simulink model "servo_system_model"  (R2021a)
settings: Solver=FixedStepAuto  StartTime=0.0  StopTime=t_end  FixedStep=dt  RelTol=1e-3
values from neighbouring files (symbols this model uses):
  A = pi/16    (= 0.196349540849)    [control_design.m]
  b1 = 0.005    [simulation.m]
  b2 = 3.7e-6    (= 3.7e-06)    [simulation.m]
  dt = 1e-4    (= 0.0001)    [parameters.m]    (also in simulation.m)
  J1 = J_barra(1)/N1^2    [simulation.m]
  J2 = J_barra(2)/N2^2    [simulation.m]
  K_sensor = 12/(pi/4)    (= 15.2788745368)    [control_design.m]    (also in parameters.m; simulation.m)
  Kb1 = 0.018    [simulation.m]
  Kb2 = 0.0145    [simulation.m]
  Kd1 = 0    [simulation.m]
  Kd2 = 0    [simulation.m]
  Ki2 = 0    [simulation.m]
  Kp1 = 1, Ki1 = 0    [simulation.m]
  Kp2 = 1    [simulation.m]
  Kt1 = 0.018    [simulation.m]
  Kt2 = 0.0145    [simulation.m]
  La1 = 2.93e-3    (= 0.00293)    [simulation.m]
  La2 = 0.42e-3    (= 0.00042)    [simulation.m]
  m = p(1)    [control_design.m]
  mode = 1    [simulation.m]
  N = 5    [parameters.m]
  N1 = 5    [simulation.m]
  N2 = 15    [simulation.m]
  Ra1 = 0.89    [simulation.m]
  Ra2 = 0.7    [simulation.m]
  s = tf('s')    [control_design.m]
  sampling = 1    [simulation.m]
  theta1_ini = theta_m(1,1)    [parameters.m]    (also in simulation.m = -1.57079632679)
  theta2_ini = theta_m(2,1)    [parameters.m]    (also in simulation.m = 0)
undefined symbols (not defined in the file or in its folder): angle_ini, displacement, home, K, Ki1, L1, L2, m1, m2, phi, X, Y, Z
libraries: sm_lib x9, fl_lib x7, nesl_utility x7, ee_lib x5, pid_lib x3, simulink x1
settings Model: Creator=Juan_Cerquera  LastModifiedBy=Sebastian

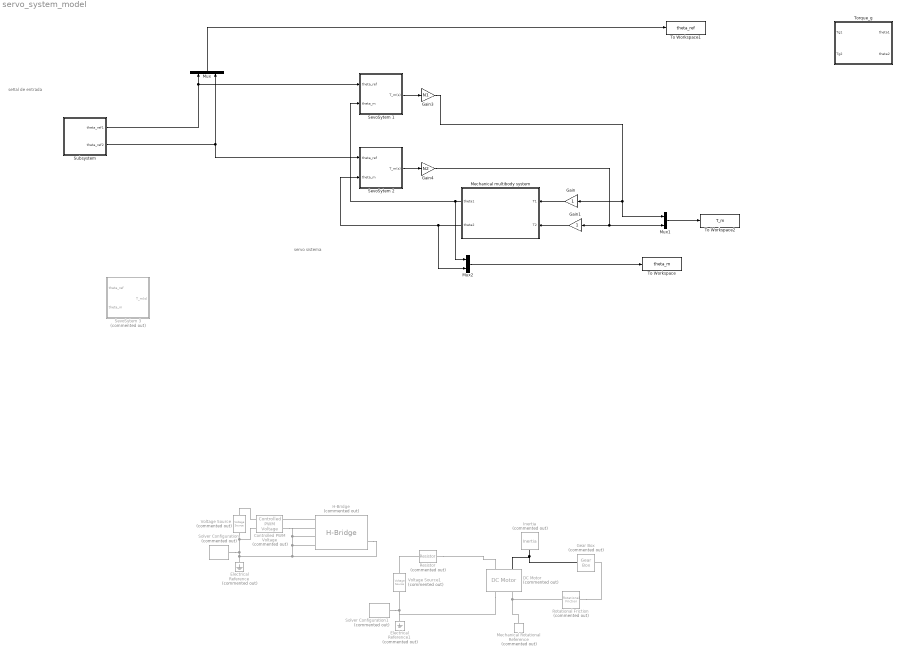
== system servo_system_model ==
  note: servo sistema
  note: señal de entrada
  Controlled PWM Voltage : ee_lib/Integrated Circuits/Controlled PWM Voltage  Commented=on  F=1000 Hz  TD=0 s  pulse_width_offset=0 s  pulse_min=0 s  Vmin=0 V  Vmax=5 V  Vm=5 V  pwm_or_av=2  event_type=1  sample_time=1e-6 s  u_min=0  u_max=1
  DC Motor : ee_lib/Electromechanical/Brushed Motors/DC Motor  Commented=on  field_option=ee.enum.field_option.pm  Rf=100 Ohm  Lf=1 H  Laf=0.15 H  If0=0 A  parameterization=ee.enum.dcparam_option.circuit_param  Ra=3.9 Ohm  La=12e-6 H  emf_or_torque=ee.enum.emf_or_torque.kv  Kv=0.072e-3 V/rpm  Ki=6.876e-4 N*m/A  T_stall=0.24e-3 N*m  w_max=19100 rpm  w_rated=15000 rpm  P_rated=0.08 W  V_rated=1.5 V  J=0.01 g*cm^2  lam_param=ee.enum.lam_param.damping  lam=0 N*m/(rad/s)  i_noload=0 A  V_i_noload=1.5 V  speed0=0 rpm  enable_fault_armature=ee.enum.faults.faultEnable.no  rev_faulted=1 / 3  G_faulted_armature=1e-5 S  fault_trigger_armature=ee.enum.faults.faultTrigger.temporal  t_fault_armature=1 s  max_permissible_current_armature=inf A  t_fail_on_current_armature=1 s  enable_fault_field=ee.enum.faults.faultEnable.no  G_faulted_field=1e-5 S  fault_trigger_field=ee.enum.faults.faultTrigger.temporal  t_fault_field=1 s  max_permissible_current_field=inf A  t_fail_on_current_field=1 s  fault_action=ee.enum.faults.faultAction.none  alpha=3.93e-3 1/K  Tmeas=25 degC  thermal_mass=100 J/K  initial_temperature=25 degC
  Electrical Reference : fl_lib/Electrical/Electrical Elements/Electrical Reference  Commented=on
  Electrical Reference1 : fl_lib/Electrical/Electrical Elements/Electrical Reference  Commented=on
  Gain : Gain
  Gain1 : Gain
  Gain3 : Gain  Gain=N1
  Gain4 : Gain  Gain=N2
  Gear Box : fl_lib/Mechanical/Mechanisms/Gear Box  Commented=on  ratio=5  t_in_specify=off  t_in_priority=None  t_in=0 N*m  t_in_nominal_specify=off  t_in_nominal_unit=N*m  t_in_nominal_value=1  t_out_specify=off  t_out_priority=None  t_out=0 N*m  t_out_nominal_specify=off  t_out_nominal_unit=N*m  t_out_nominal_value=1
  H-Bridge : ee_lib/Semiconductors & Converters/Converters/H-Bridge  Commented=on  supply_ports=ee.enum.supply_ports.hidesupply  Venable=2.5 V  Vmax=5.0 V  Vreverse=2.5 V  Vbrake=2.5 V  Vm=12 V  pwm_or_av=ee.enum.pwm_or_av.pwm  regenerative_braking_mode=ee.enum.converters.regenerative_braking_mode.depends_on_rev  discontinuous=ee.enum.current_profile.continuous  freewheeling_mode=ee.enum.converters.freewheeling_mode.one_switch_one_diode  Ron=0.1 Ohm  Don=0.05 Ohm  Goff=1e-6 S  Rload=10 Ohm  Lload=1e-5 H  F=10 kHz  thermal_mass=100 J/K  initial_temperature=298.15 K  Ron2=0.1 Ohm  Don2=0.05 Ohm  Tmeas=298.15 K  Tmeas2=398.15 K
  Inertia : fl_lib/Mechanical/Rotational Elements/Inertia  Commented=on  inertia=0.01 kg*m^2  num_ports=foundation.enum.numPorts2.one  w_specify=off  w_priority=High  w=0 rad/s  w_nominal_specify=off  w_nominal_unit=rad/s  w_nominal_value=1  t_specify=off  t_priority=None  t=0 N*m  t_nominal_specify=off  t_nominal_unit=N*m  t_nominal_value=1
  Mechanical Rotational Reference : fl_lib/Mechanical/Rotational Elements/Mechanical Rotational Reference  Commented=on
  "Mechanical multibody system " : Subsystem
  Mux : Mux  Inputs=2
  Mux1 : Mux  Inputs=2
  Mux2 : Mux  Inputs=2
  Resistor : fl_lib/Electrical/Electrical Elements/Resistor  Commented=on  R=1 Ohm  i_specify=off  i_priority=None  i=0 A  i_nominal_specify=off  i_nominal_unit=A  i_nominal_value=1  v_specify=off  v_priority=None  v=0 V  v_nominal_specify=off  v_nominal_unit=V  v_nominal_value=1
  Rotational Friction : fl_lib/Mechanical/Rotational Elements/Rotational Friction  Commented=on  brkwy_trq=25 N*m  brkwy_vel=0.1 rad/s  Col_trq=20 N*m  visc_coef=0.001 N*m/(rad/s)  w_specify=off  w_priority=None  w=0 rad/s  w_nominal_specify=off  w_nominal_unit=rad/s  w_nominal_value=1  t_specify=off  t_priority=None  t=0 N*m  t_nominal_specify=off  t_nominal_unit=N*m  t_nominal_value=1
  SevoSytem 1 : Subsystem  mask{P=Kp1, I=Ki1, D=Kd1, InitialCondition=theta1_ini, Electric=[La1 Ra1], Mechanic=[J1 b1], Kb=Kb1, Kt=Kt1, K_sensor=K_sensor}
      mask prompts: P "Simulink:masks:ProportionalP_MP"; I "Simulink:masks:IntegralI_MP"; D "Simulink:masks:DerivativeD_MP"; InitialCondition "Simulink:blkprm_prompts:AllBlksInitConds"; Electric "Electrical system Denominator"; Mechanic "Mechanical system Denominator"; Kb "Gain Kb:"; Kt "Gain Kt:"; K_sensor "Gain Sensor:"
      mask TypeOptions P: controlador/P
      mask TypeOptions I: controlador/I
      mask TypeOptions D: controlador/D
      mask TypeOptions InitialCondition: integrador/InitialCondition
      mask TypeOptions Electric: motor/Electric system/Denominator
      mask TypeOptions Mechanic: motor/Mechanic system/Denominator
      mask TypeOptions Kb: motor/kb/Gain
      mask TypeOptions Kt: motor/kt/Gain
      mask TypeOptions K_sensor: sensor/Gain
      mask DialogControl P Prompt: Proportional (P):
      mask DialogControl I Prompt: Integral (I):
      mask DialogControl D Prompt: Derivative (D):
      mask DialogControl InitialCondition Prompt: Initial conditions:
  SevoSytem 2 : Subsystem  mask{P=Kp2, I=Ki2, D=Kd2, InitialCondition=theta2_ini, Electric=[La2 Ra2], Mechanic=[J2 b2], Kb=Kb2, Kt=Kt2, K_sensor=K_sensor}
      mask prompts: P "Simulink:masks:ProportionalP_MP"; I "Simulink:masks:IntegralI_MP"; D "Simulink:masks:DerivativeD_MP"; InitialCondition "Simulink:blkprm_prompts:AllBlksInitConds"; Electric "Electrical system Denominator"; Mechanic "Mechanical system Denominator"; Kb "Gain Kb:"; Kt "Gain Kt:"; K_sensor "Gain Sensor:"
      mask TypeOptions P: controlador/P
      mask TypeOptions I: controlador/I
      mask TypeOptions D: controlador/D
      mask TypeOptions InitialCondition: integrador/InitialCondition
      mask TypeOptions Electric: motor/Electric system/Denominator
      mask TypeOptions Mechanic: motor/Mechanic system/Denominator
      mask TypeOptions Kb: motor/kb/Gain
      mask TypeOptions Kt: motor/kt/Gain
      mask TypeOptions K_sensor: sensor/Gain
      mask DialogControl P Prompt: Proportional (P):
      mask DialogControl I Prompt: Integral (I):
      mask DialogControl D Prompt: Derivative (D):
      mask DialogControl InitialCondition Prompt: Initial conditions:
  SevoSytem 3 : Subsystem  Commented=on  mask{P=Kp1, I=Ki1, D=Kd1, InitialCondition=theta1_ini, Electric=[La1 Ra1], Mechanic=[J1 b1], Kb=Kb1, Kt=Kt1, K_sensor=K_sensor}
      mask prompts: P "Simulink:masks:ProportionalP_MP"; I "Simulink:masks:IntegralI_MP"; D "Simulink:masks:DerivativeD_MP"; InitialCondition "Simulink:blkprm_prompts:AllBlksInitConds"; Electric "Electrical system Denominator"; Mechanic "Mechanical system Denominator"; Kb "Gain Kb:"; Kt "Gain Kt:"; K_sensor "Gain Sensor:"
      mask TypeOptions P: controlador/P
      mask TypeOptions I: controlador/I
      mask TypeOptions D: controlador/D
      mask TypeOptions InitialCondition: integrador/InitialCondition
      mask TypeOptions Electric: motor/Electric system/Denominator
      mask TypeOptions Mechanic: motor/Mechanic system/Denominator
      mask TypeOptions Kb: motor/kb/Gain
      mask TypeOptions Kt: motor/kt/Gain
      mask TypeOptions K_sensor: sensor/Gain
      mask DialogControl P Prompt: Proportional (P):
      mask DialogControl I Prompt: Integral (I):
      mask DialogControl D Prompt: Derivative (D):
      mask DialogControl InitialCondition Prompt: Initial conditions:
  Solver Configuration : nesl_utility/Solver Configuration  Commented=on  PhysicalDomain=network_engine_domain  SubClassName=solver  LeftPortType=input  RightPortType=generic  Tones=[]  Harmonics=[]  SimulateNoise=off  Profile=off  UseLocalSampling=off  EnableSwitchedLinearOptims=on  FrequencyDomain=off  UseCCode=off  RelTol=0.001  AbsTol=1e-06  MinStep=1e-09  ToWorkspace=off  RevertToSquareIcSolve=off  NumHomotopyIterations=100  PhasorMode=off  PhasorModeNumHarmonics=1  DoDC=off  ResidualTolerance=1e-09  UseLocalSolver=off  LocalSolverChoice=NE_BACKWARD_EULER_ADVANCER  LocalSolverSampleTime=0.001  DoFixedCost=off  MaxNonlinIter=3  MaxModeIter=2  ComputeImpulses=off  ImpulseIterations=2  LinearAlgebra=auto  EquationFormulation=NE_TIME_EF  DelaysMemoryBudget=1024  AutomaticFiltering=on  FilteringTimeConstant=0.001  PartitionStorageMethod=AS_NEEDED  PartitionMemoryBudget=1024  PartitionMethod=ROBUST
      settings: SourceProductBaseCode=PW,SS
  Solver Configuration1 : nesl_utility/Solver Configuration  Commented=on  PhysicalDomain=network_engine_domain  SubClassName=solver  LeftPortType=input  RightPortType=generic  Tones=[]  Harmonics=[]  SimulateNoise=off  Profile=off  UseLocalSampling=off  EnableSwitchedLinearOptims=on  FrequencyDomain=off  UseCCode=off  RelTol=0.001  AbsTol=1e-06  MinStep=1e-09  ToWorkspace=off  RevertToSquareIcSolve=off  NumHomotopyIterations=100  PhasorMode=off  PhasorModeNumHarmonics=1  DoDC=off  ResidualTolerance=1e-09  UseLocalSolver=off  LocalSolverChoice=NE_BACKWARD_EULER_ADVANCER  LocalSolverSampleTime=0.001  DoFixedCost=off  MaxNonlinIter=3  MaxModeIter=2  ComputeImpulses=off  ImpulseIterations=2  LinearAlgebra=auto  EquationFormulation=NE_TIME_EF  DelaysMemoryBudget=1024  AutomaticFiltering=on  FilteringTimeConstant=0.001  PartitionStorageMethod=AS_NEEDED  PartitionMemoryBudget=1024  PartitionMethod=ROBUST
      settings: SourceProductBaseCode=PW,SS
  Subsystem : Subsystem  mask{angle_ini=angle_ini, K=K, phi=phi, A=A}
      mask prompts: angle_ini "angulo inicial"; K "factor de escala"; phi "desface"; A "factor de estilizado"
      mask TypeOptions angle_ini: angle_ini/Value
      mask TypeOptions K: K/Value
      mask TypeOptions phi: phi/Value
      mask TypeOptions A: A/Value
  To Workspace : ToWorkspace  VariableName=theta_m  SaveFormat=Timeseries  SampleTime=sampling*dt
  To Workspace1 : ToWorkspace  VariableName=theta_ref  SaveFormat=Timeseries  SampleTime=sampling*dt
  To Workspace2 : ToWorkspace  VariableName=T_m  SaveFormat=Timeseries  SampleTime=sampling*dt
  Torque_g : MATLAB Function  TreatAsAtomicUnit=on
  Voltage Source : ee_lib/Sources/Voltage Source  Commented=on  dc_voltage=12 V  ac_voltage=0 V  ac_shift=0 rad  ac_frequency=60 Hz  noise_mode=0  PSD=0 V^2/Hz  repeatability=1  auto_seed=3529265616  user_seed=0  sample_time=1e-3 s  i_specify=off  i_priority=None  i=0 A  i_nominal_specify=off  i_nominal_unit=A  i_nominal_value=1  v_specify=off  v_priority=None  v=0 V  v_nominal_specify=off  v_nominal_unit=V  v_nominal_value=1
  Voltage Source1 : ee_lib/Sources/Voltage Source  Commented=on  dc_voltage=12 V  ac_voltage=0 V  ac_shift=0 rad  ac_frequency=60 Hz  noise_mode=0  PSD=0 V^2/Hz  repeatability=1  auto_seed=1078396959  user_seed=0  sample_time=1e-3 s  i_specify=off  i_priority=None  i=0 A  i_nominal_specify=off  i_nominal_unit=A  i_nominal_value=1  v_specify=off  v_priority=None  v=0 V  v_nominal_specify=off  v_nominal_unit=V  v_nominal_value=1
  wires:
  Subsystem/2(theta_ref2) -> Mux/2, SevoSytem 2/1(theta_ref)
  Subsystem/1(theta_ref1) -> Mux/1, SevoSytem 1/1(theta_ref)
  Mux1/1 -> To Workspace2/1
  Mux2/1 -> To Workspace/1
  Mux/1 -> To Workspace1/1
  "Mechanical multibody system "/1(theta1) -> Mux2/1, SevoSytem 1/2(theta_m)
  "Mechanical multibody system "/2(theta2) -> Mux2/2, SevoSytem 2/2(theta_m)
  SevoSytem 1/1(T_m(s)) -> Gain3/1
  Gain3/1 -> Gain/1, Mux1/1
  Gain4/1 -> Gain1/1, Mux1/2
  SevoSytem 2/1(T_m(s)) -> Gain4/1
  Gain/1 -> "Mechanical multibody system "/1(T1)
  Gain1/1 -> "Mechanical multibody system "/2(T2)
  connections:
  Electrical Reference/LConn1 -- H-Bridge/RConn2 -- H-Bridge/LConn4 -- H-Bridge/LConn3 -- H-Bridge/LConn2 -- Controlled PWM Voltage/RConn2 -- Solver Configuration/RConn1 -- Controlled PWM Voltage/LConn2 -- Voltage Source/RConn1
  Controlled PWM Voltage/LConn1 -- Voltage Source/LConn1
  H-Bridge/LConn1 -- Controlled PWM Voltage/RConn1
  Inertia/LConn1 -- Gear Box/LConn1 -- DC Motor/LConn2
  Mechanical Rotational Reference/LConn1 -- Rotational Friction/RConn1 -- DC Motor/RConn2
  Resistor/RConn1 -- DC Motor/LConn1
  Rotational Friction/LConn1 -- Gear Box/RConn1
  Solver Configuration1/RConn1 -- DC Motor/RConn1 -- Electrical Reference1/LConn1 -- Voltage Source1/RConn1
  Voltage Source1/LConn1 -- Resistor/LConn1

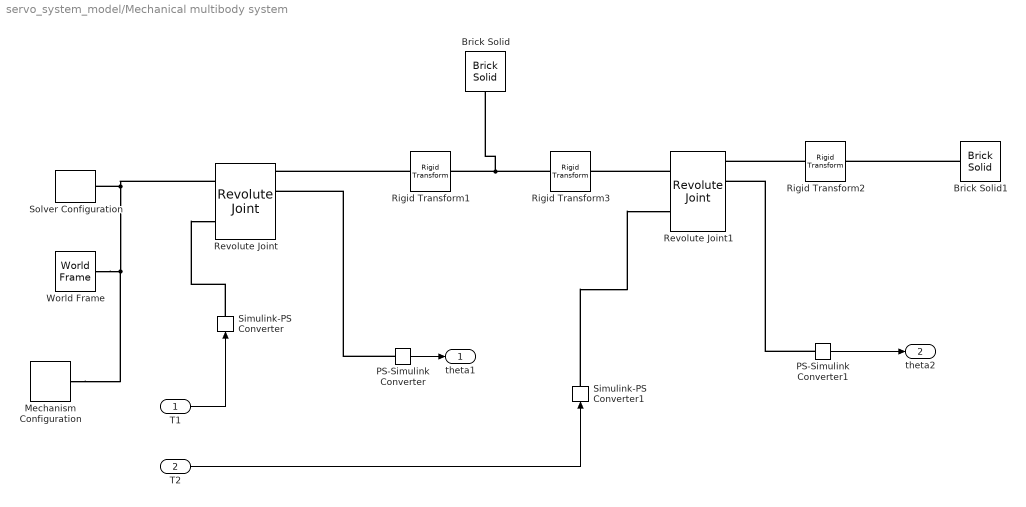
== system servo_system_model/Mechanical multibody system  ==
  T1 : Inport
  T2 : Inport  Port=2
  Brick Solid : sm_lib/Body Elements/Brick Solid  GraphicAmbientColor=[0.15 0.15 0.15 1.0]  BasedOnType=Density  BrickDimensions=[L1 1 1]  BrickDimensionUnits=cm  CenterOfMass=[0 0 0]  CenterOfMassUnits=m  GraphicDiffuseColor=[0 0 1]  Density=1000  DensityUnits=kg/m^3  DoExposeReferenceFrame=on  GraphicEmissiveColor=[0.0 0.0 0.0 1.0]  ExportEntireGeometry=off  SerializedFrames=<Frames/>  MarkerShape=Sphere  MarkerSize=10  GraphicType=FromGeometry  InertiaType=PointMass  Mass=m1/N1  MassUnits=kg  MomentsOfInertia=[1 1 1]  MomentsOfInertiaUnits=kg*m^2  GraphicOpacity=1.0  ProductsOfInertia=[0 0 0]  ProductsOfInertiaUnits=kg*m^2  GraphicShininess=75  GraphicSpecularColor=[0.5 0.5 0.5 1.0]  GraphicVisPropType=SimpleVisualProperties
  Brick Solid1 : sm_lib/Body Elements/Brick Solid  GraphicAmbientColor=[0.15 0.15 0.15 1.0]  BasedOnType=Density  BrickDimensions=[L2 1 1]  BrickDimensionUnits=cm  CenterOfMass=[0 0 0]  CenterOfMassUnits=m  GraphicDiffuseColor=[1 0 0]  Density=1000  DensityUnits=kg/m^3  DoExposeReferenceFrame=on  GraphicEmissiveColor=[0.0 0.0 0.0 1.0]  ExportEntireGeometry=off  SerializedFrames=<Frames/>  MarkerShape=Sphere  MarkerSize=10  GraphicType=FromGeometry  InertiaType=PointMass  Mass=m2/N2  MassUnits=kg  MomentsOfInertia=[1 1 1]  MomentsOfInertiaUnits=kg*m^2  GraphicOpacity=1.0  ProductsOfInertia=[0 0 0]  ProductsOfInertiaUnits=kg*m^2  GraphicShininess=75  GraphicSpecularColor=[0.5 0.5 0.5 1.0]  GraphicVisPropType=SimpleVisualProperties
  Mechanism Configuration : sm_lib/Utilities/Mechanism Configuration  UniformGravity=Constant  GravityVector=[0 -9.80665 0]  GravityVectorUnits=m/s^2  GravityUnits=m/s^2  LinearizationDelta=0.001  JointModeTransitionNonlinearIterations=2
  PS-Simulink Converter : nesl_utility/PS-Simulink Converter  PhysicalDomain=network_engine_domain  SubClassName=ps_output  LeftPortType=input  RightPortType=output  PseudoPeriodic=off  Frequencies=[]  Unit=inherit  AffineConversion=off
      settings: SourceProductBaseCode=PW,SS
  PS-Simulink Converter1 : nesl_utility/PS-Simulink Converter  PhysicalDomain=network_engine_domain  SubClassName=ps_output  LeftPortType=input  RightPortType=output  PseudoPeriodic=off  Frequencies=[]  Unit=inherit  AffineConversion=off
      settings: SourceProductBaseCode=PW,SS
  Revolute Joint : sm_lib/Joints/Revolute Joint  JointMode=Normal  SenseConstraintForce=off  SenseConstraintForceX=off  SenseConstraintForceY=off  SenseConstraintForceZ=off  SenseConstraintTorque=off  SenseConstraintTorqueX=off  SenseConstraintTorqueY=off  SenseConstraintTorqueZ=off  SenseTotalForce=off  SenseTotalForceX=off  SenseTotalForceY=off  SenseTotalForceZ=off  SenseTotalTorque=off  SenseTotalTorqueX=off  SenseTotalTorqueY=off  SenseTotalTorqueZ=off  CompositeWrenchDir=FollowerOnBase  CompositeWrenchFrame=BaseFrame  EquilibriumPosition=0  EquilibriumPositionUnits=deg  SpringStiffness=0  SpringStiffnessUnits=N*m/deg  DampingCoefficient=0  DampingCoefficientUnits=N*m/(deg/s)  TorqueActuationMode=InputTorque  MotionActuationMode=ComputedMotion  SensePosition=on  SenseVelocity=on  SenseAcceleration=on  SenseTorqueForce=off  SenseLowerLimitTorqueForce=off  SenseUpperLimitTorqueForce=off  LowerLimitSpecify=off  LowerLimitBound=-90  LowerLimitBoundUnits=deg  LowerLimitStiffness=1e4  LowerLimitStiffnessUnits=N*m/deg  LowerLimitDamping=10  LowerLimitDampingUnits=N*m/(deg/s)  LowerLimitTransitionRegionWidth=0.1  LowerLimitTransitionRegionWidthUnits=deg  UpperLimitSpecify=off  UpperLimitBound=90  UpperLimitBoundUnits=deg  UpperLimitStiffness=1e4  UpperLimitStiffnessUnits=N*m/deg  UpperLimitDamping=10  UpperLimitDampingUnits=N*m/(deg/s)  UpperLimitTransitionRegionWidth=0.1  UpperLimitTransitionRegionWidthUnits=deg  PositionTargetSpecify=off  PositionTargetPriority=High  PositionTargetValue=0  PositionTargetValueUnits=deg  VelocityTargetSpecify=off  VelocityTargetPriority=High  VelocityTargetValue=0  VelocityTargetValueUnits=deg/s
  Revolute Joint1 : sm_lib/Joints/Revolute Joint  JointMode=Normal  SenseConstraintForce=off  SenseConstraintForceX=off  SenseConstraintForceY=off  SenseConstraintForceZ=off  SenseConstraintTorque=off  SenseConstraintTorqueX=off  SenseConstraintTorqueY=off  SenseConstraintTorqueZ=off  SenseTotalForce=off  SenseTotalForceX=off  SenseTotalForceY=off  SenseTotalForceZ=off  SenseTotalTorque=off  SenseTotalTorqueX=off  SenseTotalTorqueY=off  SenseTotalTorqueZ=off  CompositeWrenchDir=FollowerOnBase  CompositeWrenchFrame=BaseFrame  EquilibriumPosition=0  EquilibriumPositionUnits=deg  SpringStiffness=0  SpringStiffnessUnits=N*m/deg  DampingCoefficient=0  DampingCoefficientUnits=N*m/(deg/s)  TorqueActuationMode=InputTorque  MotionActuationMode=ComputedMotion  SensePosition=on  SenseVelocity=on  SenseAcceleration=on  SenseTorqueForce=off  SenseLowerLimitTorqueForce=off  SenseUpperLimitTorqueForce=off  LowerLimitSpecify=off  LowerLimitBound=-90  LowerLimitBoundUnits=deg  LowerLimitStiffness=1e4  LowerLimitStiffnessUnits=N*m/deg  LowerLimitDamping=10  LowerLimitDampingUnits=N*m/(deg/s)  LowerLimitTransitionRegionWidth=0.1  LowerLimitTransitionRegionWidthUnits=deg  UpperLimitSpecify=off  UpperLimitBound=90  UpperLimitBoundUnits=deg  UpperLimitStiffness=1e4  UpperLimitStiffnessUnits=N*m/deg  UpperLimitDamping=10  UpperLimitDampingUnits=N*m/(deg/s)  UpperLimitTransitionRegionWidth=0.1  UpperLimitTransitionRegionWidthUnits=deg  PositionTargetSpecify=off  PositionTargetPriority=High  PositionTargetValue=0  PositionTargetValueUnits=deg  VelocityTargetSpecify=off  VelocityTargetPriority=High  VelocityTargetValue=0  VelocityTargetValueUnits=deg/s
  Rigid Transform1 : sm_lib/Frames and Transforms/Rigid Transform  TranslationMethod=StandardAxis  TranslationStandardOffset=L1/2  TranslationLengthUnit=cm  TranslationStandardAxis=+X  TranslationCartesianOffset=[0 0 0]  TranslationROffset=0  TranslationROffsetUnits=m  TranslationZOffset=0  TranslationZOffsetUnits=m  TranslationThetaOffset=0  TranslationThetaOffsetUnits=deg  RotationMethod=None  RotationAngleUnits=deg  RotationStandardAxis=+Z  RotationAngle=0.0  RotationArbitraryAxis=[0 0 1]  FollAlignAxisA=+X  BaseAlignAxisA=+Y  FollAlignAxisB=+Y  BaseAlignAxisB=+Z  RotationSequenceAxes=FollowerAxes  RotationSequence=XYX  RotationSequenceAngles=[0 0 0]  RotationSequenceAnglesUnits=deg  RotationMatrix=[1 0 0; 0 1 0; 0 0 1]
  Rigid Transform2 : sm_lib/Frames and Transforms/Rigid Transform  TranslationMethod=StandardAxis  TranslationStandardOffset=L2/2  TranslationLengthUnit=cm  TranslationStandardAxis=+X  TranslationCartesianOffset=[0 0 0]  TranslationROffset=0  TranslationROffsetUnits=m  TranslationZOffset=0  TranslationZOffsetUnits=m  TranslationThetaOffset=0  TranslationThetaOffsetUnits=deg  RotationMethod=None  RotationAngleUnits=deg  RotationStandardAxis=+Z  RotationAngle=0.0  RotationArbitraryAxis=[0 0 1]  FollAlignAxisA=+X  BaseAlignAxisA=+Y  FollAlignAxisB=+Y  BaseAlignAxisB=+Z  RotationSequenceAxes=FollowerAxes  RotationSequence=XYX  RotationSequenceAngles=[0 0 0]  RotationSequenceAnglesUnits=deg  RotationMatrix=[1 0 0; 0 1 0; 0 0 1]
  Rigid Transform3 : sm_lib/Frames and Transforms/Rigid Transform  TranslationMethod=StandardAxis  TranslationStandardOffset=L1/2  TranslationLengthUnit=cm  TranslationStandardAxis=+X  TranslationCartesianOffset=[0 0 0]  TranslationROffset=0  TranslationROffsetUnits=m  TranslationZOffset=0  TranslationZOffsetUnits=m  TranslationThetaOffset=0  TranslationThetaOffsetUnits=deg  RotationMethod=None  RotationAngleUnits=deg  RotationStandardAxis=+Z  RotationAngle=0.0  RotationArbitraryAxis=[0 0 1]  FollAlignAxisA=+X  BaseAlignAxisA=+Y  FollAlignAxisB=+Y  BaseAlignAxisB=+Z  RotationSequenceAxes=FollowerAxes  RotationSequence=XYX  RotationSequenceAngles=[0 0 0]  RotationSequenceAnglesUnits=deg  RotationMatrix=[1 0 0; 0 1 0; 0 0 1]
  Simulink-PS Converter : nesl_utility/Simulink-PS Converter  PhysicalDomain=network_engine_domain  SubClassName=ps_input  LeftPortType=input  RightPortType=output  PseudoPeriodic=off  Frequencies=[]  NoiseDistribution=none  NoiseParameters=[]  Unit=N*m  AffineConversion=off  FilteringAndDerivatives=filter  SimscapeFilterOrder=2  InputFilterTimeConstant=0.001  UdotUserProvided=0
      settings: SourceProductBaseCode=PW,SS
  Simulink-PS Converter1 : nesl_utility/Simulink-PS Converter  PhysicalDomain=network_engine_domain  SubClassName=ps_input  LeftPortType=input  RightPortType=output  PseudoPeriodic=off  Frequencies=[]  NoiseDistribution=none  NoiseParameters=[]  Unit=N*m  AffineConversion=off  FilteringAndDerivatives=filter  SimscapeFilterOrder=2  InputFilterTimeConstant=0.001  UdotUserProvided=0
      settings: SourceProductBaseCode=PW,SS
  Solver Configuration : nesl_utility/Solver Configuration  PhysicalDomain=network_engine_domain  SubClassName=solver  LeftPortType=input  RightPortType=generic  Tones=[]  Harmonics=[]  SimulateNoise=off  Profile=off  UseLocalSampling=off  EnableSwitchedLinearOptims=on  FrequencyDomain=off  UseCCode=off  RelTol=0.001  AbsTol=1e-06  MinStep=1e-09  ToWorkspace=off  RevertToSquareIcSolve=off  NumHomotopyIterations=100  PhasorMode=off  PhasorModeNumHarmonics=1  DoDC=off  ResidualTolerance=1e-09  UseLocalSolver=off  LocalSolverChoice=NE_BACKWARD_EULER_ADVANCER  LocalSolverSampleTime=0.001  DoFixedCost=off  MaxNonlinIter=3  MaxModeIter=2  ComputeImpulses=off  ImpulseIterations=2  LinearAlgebra=Sparse  EquationFormulation=NE_TIME_EF  DelaysMemoryBudget=1024  AutomaticFiltering=on  FilteringTimeConstant=0.001  PartitionStorageMethod=AS_NEEDED  PartitionMemoryBudget=1024  PartitionMethod=FAST
      settings: SourceProductBaseCode=PW,SS
  World Frame : sm_lib/Frames and Transforms/World Frame
  theta1 : Outport
  theta2 : Outport  Port=2
  wires:
  T1/1 -> Simulink-PS Converter/1
  T2/1 -> Simulink-PS Converter1/1
  PS-Simulink Converter1/1 -> theta2/1
  PS-Simulink Converter/1 -> theta1/1
  connections:
  Revolute Joint1/LConn1 -- Rigid Transform3/RConn1
  World Frame/RConn1 -- Revolute Joint/LConn1 -- Solver Configuration/RConn1 -- Mechanism Configuration/RConn1
  Brick Solid1/RConn1 -- Rigid Transform2/RConn1
  Rigid Transform3/LConn1 -- Brick Solid/RConn1 -- Rigid Transform1/RConn1
  Rigid Transform1/LConn1 -- Revolute Joint/RConn1
  Rigid Transform2/LConn1 -- Revolute Joint1/RConn1
  Simulink-PS Converter/RConn1 -- Revolute Joint/LConn2
  Simulink-PS Converter1/RConn1 -- Revolute Joint1/LConn2
  PS-Simulink Converter1/LConn1 -- Revolute Joint1/RConn2
  PS-Simulink Converter/LConn1 -- Revolute Joint/RConn2

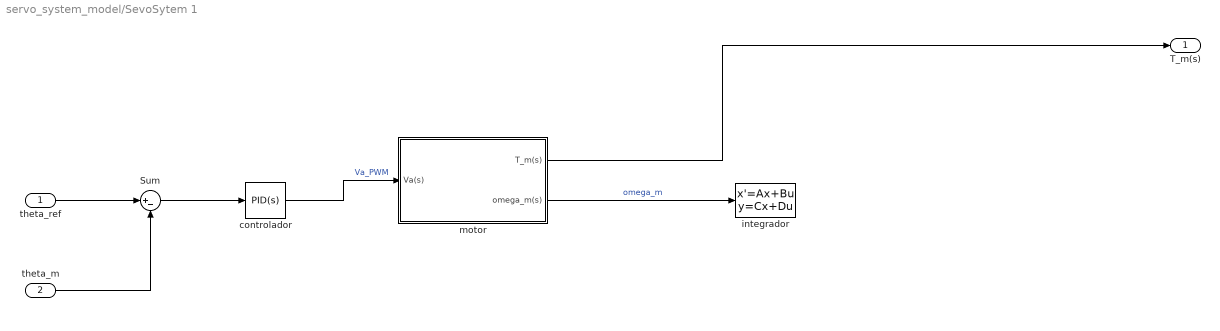
== system servo_system_model/SevoSytem 1 ==
  theta_ref : Inport
  theta_m : Inport  Port=2
  Sum : Sum  Inputs=|+-
  controlador : pid_lib/PID Controller  Controller=PID  Form=Parallel  TimeDomain=Continuous-time  UseExternalTs=off  SampleTime=-1  IntegratorMethod=Forward Euler  FilterMethod=Forward Euler  ControllerParametersSource=internal  P=P  I=I  D=D  UseFilter=on  N=100  TunerSelectOption=Transfer Function Based (PID Tuner App)  InitialConditionSource=internal  InitialConditionForIntegrator=0  InitialConditionForFilter=0  DifferentiatorICPrevScaledInput=0  ExternalReset=none  TrackingMode=off  Kt=1  LimitOutput=off  SatLimitsSource=internal  UpperSaturationLimit=inf  LowerSaturationLimit=-inf  LinearizeAsGain=on  AntiWindupMode=none  Kb=1  POutMin=[]  POutMax=[]  IOutMin=[]  IOutMax=[]  DOutMin=[]  DOutMax=[]  NOutMin=[]  NOutMax=[]  SumOutMin=[]  SumOutMax=[]  SaturationOutMin=[]  SaturationOutMax=[]  PParamMin=[]  PParamMax=[]  IParamMin=[]  IParamMax=[]  DParamMin=[]  DParamMax=[]  NParamMin=[]  NParamMax=[]  KbParamMin=[]  KbParamMax=[]  KtParamMin=[]  KtParamMax=[]  KbOutMin=[]  KbOutMax=[]  KtOutMin=[]  KtOutMax=[]  IntegratorOutMin=[]  IntegratorOutMax=[]  FilterOutMin=[]  FilterOutMax=[]  SumI1OutMin=[]  SumI1OutMax=[]  SumI2OutMin=[]  SumI2OutMax=[]  SumI3OutMin=[]  SumI3OutMax=[]  SumI4OutMin=[]  SumI4OutMax=[]  SumDOutMin=[]  SumDOutMax=[]  DifferentiatorOutMin=[]  DifferentiatorOutMax=[]  FilterDiffOutCoefMin=[]  FilterDiffOutCoefMax=[]  ReciprocalOutMin=[]  ReciprocalOutMax=[]  SumDenOutMin=[]  SumDenOutMax=[]  SumNumOutMin=[]  SumNumOutMax=[]  DivideOutMin=[]  DivideOutMax=[]  UdiffTsProdOutMin=[]  UdiffTsProdOutMax=[]  NTsProdOutMin=[]  NTsProdOutMax=[]  UintegralTsProdOutMin=[]  UintegralTsProdOutMax=[]  UngainTsProdOutMin=[]  UngainTsProdOutMax=[]  IntegratorContinuousStateAttributes=''  IntegratorStateMustResolveToSignalObject=off  IntegratorRTWStateStorageClass=Auto  FilterContinuousStateAttributes=''  FilterStateMustResolveToSignalObject=off  FilterRTWStateStorageClass=Auto  ParallelPVariant=InternalParameters  IdealPVariant=Disabled  IVariant=InternalParameters  DVariant=InternalParameters  IntegratorVariant=Continuous  SatVariant=Disabled  AWVariant=Passthrough  PCopyVariant=Disabled  TRVariant=Disabled  FdbkBlocksVariant=Forward  IdealPFdbkVariant=Disabled  SatFdbkVariant=Disabled  DerivativeFilterVariant=ContFilter  NVariant=InternalParameters  NCopyVariant=Disabled  FilterICVariant=InternalICsFilter  IntegratorICVariant=InternalICs  ExternalResetVariant=Disabled  TRSumVariant=Passthrough  SumFdbkVariant=Disabled  SumVariant=Sum_PID  TsampFilterVariant=InternalTs  TsampNgainVariant=Passthrough  TsampIntegralVariant=Passthrough  ExternalSaturationOutDataTypeStr=Inherit: Same as second input
  integrador : StateSpace  A=0  D=0  InitialCondition=InitialCondition
  motor : Subsystem
  T_m(s) : Outport
  wires:
  motor/2(omega_m(s)) -> integrador/1  "omega_m"
  Sum/1 -> controlador/1
  controlador/1 -> motor/1(Va(s))  "Va_PWM"
  theta_ref/1 -> Sum/1
  motor/1(T_m(s)) -> T_m(s)/1
  theta_m/1 -> Sum/2

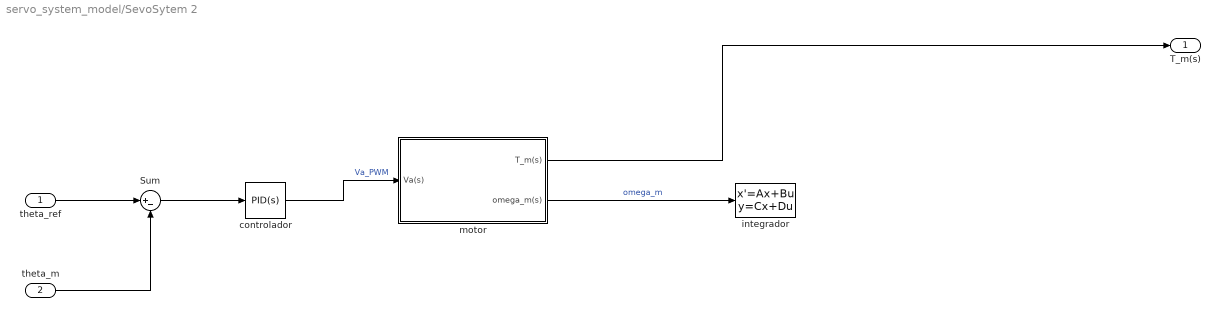
== system servo_system_model/SevoSytem 2 ==
  theta_ref : Inport
  theta_m : Inport  Port=2
  Sum : Sum  Inputs=|+-
  controlador : pid_lib/PID Controller  Controller=PID  Form=Parallel  TimeDomain=Continuous-time  UseExternalTs=off  SampleTime=-1  IntegratorMethod=Forward Euler  FilterMethod=Forward Euler  ControllerParametersSource=internal  P=P  I=I  D=D  UseFilter=on  N=100  TunerSelectOption=Transfer Function Based (PID Tuner App)  InitialConditionSource=internal  InitialConditionForIntegrator=0  InitialConditionForFilter=0  DifferentiatorICPrevScaledInput=0  ExternalReset=none  TrackingMode=off  Kt=1  LimitOutput=off  SatLimitsSource=internal  UpperSaturationLimit=inf  LowerSaturationLimit=-inf  LinearizeAsGain=on  AntiWindupMode=none  Kb=1  POutMin=[]  POutMax=[]  IOutMin=[]  IOutMax=[]  DOutMin=[]  DOutMax=[]  NOutMin=[]  NOutMax=[]  SumOutMin=[]  SumOutMax=[]  SaturationOutMin=[]  SaturationOutMax=[]  PParamMin=[]  PParamMax=[]  IParamMin=[]  IParamMax=[]  DParamMin=[]  DParamMax=[]  NParamMin=[]  NParamMax=[]  KbParamMin=[]  KbParamMax=[]  KtParamMin=[]  KtParamMax=[]  KbOutMin=[]  KbOutMax=[]  KtOutMin=[]  KtOutMax=[]  IntegratorOutMin=[]  IntegratorOutMax=[]  FilterOutMin=[]  FilterOutMax=[]  SumI1OutMin=[]  SumI1OutMax=[]  SumI2OutMin=[]  SumI2OutMax=[]  SumI3OutMin=[]  SumI3OutMax=[]  SumI4OutMin=[]  SumI4OutMax=[]  SumDOutMin=[]  SumDOutMax=[]  DifferentiatorOutMin=[]  DifferentiatorOutMax=[]  FilterDiffOutCoefMin=[]  FilterDiffOutCoefMax=[]  ReciprocalOutMin=[]  ReciprocalOutMax=[]  SumDenOutMin=[]  SumDenOutMax=[]  SumNumOutMin=[]  SumNumOutMax=[]  DivideOutMin=[]  DivideOutMax=[]  UdiffTsProdOutMin=[]  UdiffTsProdOutMax=[]  NTsProdOutMin=[]  NTsProdOutMax=[]  UintegralTsProdOutMin=[]  UintegralTsProdOutMax=[]  UngainTsProdOutMin=[]  UngainTsProdOutMax=[]  IntegratorContinuousStateAttributes=''  IntegratorStateMustResolveToSignalObject=off  IntegratorRTWStateStorageClass=Auto  FilterContinuousStateAttributes=''  FilterStateMustResolveToSignalObject=off  FilterRTWStateStorageClass=Auto  ParallelPVariant=InternalParameters  IdealPVariant=Disabled  IVariant=InternalParameters  DVariant=InternalParameters  IntegratorVariant=Continuous  SatVariant=Disabled  AWVariant=Passthrough  PCopyVariant=Disabled  TRVariant=Disabled  FdbkBlocksVariant=Forward  IdealPFdbkVariant=Disabled  SatFdbkVariant=Disabled  DerivativeFilterVariant=ContFilter  NVariant=InternalParameters  NCopyVariant=Disabled  FilterICVariant=InternalICsFilter  IntegratorICVariant=InternalICs  ExternalResetVariant=Disabled  TRSumVariant=Passthrough  SumFdbkVariant=Disabled  SumVariant=Sum_PID  TsampFilterVariant=InternalTs  TsampNgainVariant=Passthrough  TsampIntegralVariant=Passthrough  ExternalSaturationOutDataTypeStr=Inherit: Same as second input
  integrador : StateSpace  A=0  D=0  InitialCondition=InitialCondition
  motor : Subsystem
  T_m(s) : Outport
  wires:
  motor/2(omega_m(s)) -> integrador/1  "omega_m"
  Sum/1 -> controlador/1
  controlador/1 -> motor/1(Va(s))  "Va_PWM"
  theta_ref/1 -> Sum/1
  motor/1(T_m(s)) -> T_m(s)/1
  theta_m/1 -> Sum/2

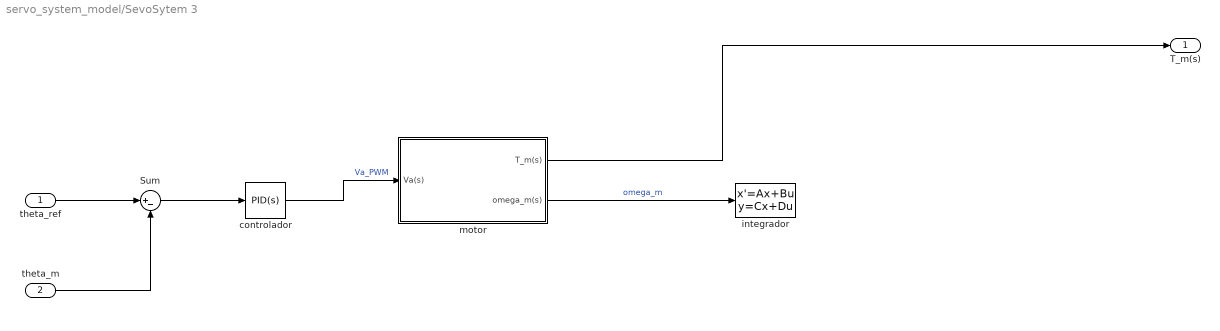
== system servo_system_model/SevoSytem 3 ==
  theta_ref : Inport
  theta_m : Inport  Port=2
  Sum : Sum  Inputs=|+-
  controlador : pid_lib/PID Controller  Controller=PID  Form=Parallel  TimeDomain=Continuous-time  UseExternalTs=off  SampleTime=-1  IntegratorMethod=Forward Euler  FilterMethod=Forward Euler  ControllerParametersSource=internal  P=P  I=I  D=D  UseFilter=on  N=100  TunerSelectOption=Transfer Function Based (PID Tuner App)  InitialConditionSource=internal  InitialConditionForIntegrator=0  InitialConditionForFilter=0  DifferentiatorICPrevScaledInput=0  ExternalReset=none  TrackingMode=off  Kt=1  LimitOutput=off  SatLimitsSource=internal  UpperSaturationLimit=inf  LowerSaturationLimit=-inf  LinearizeAsGain=on  AntiWindupMode=none  Kb=1  POutMin=[]  POutMax=[]  IOutMin=[]  IOutMax=[]  DOutMin=[]  DOutMax=[]  NOutMin=[]  NOutMax=[]  SumOutMin=[]  SumOutMax=[]  SaturationOutMin=[]  SaturationOutMax=[]  PParamMin=[]  PParamMax=[]  IParamMin=[]  IParamMax=[]  DParamMin=[]  DParamMax=[]  NParamMin=[]  NParamMax=[]  KbParamMin=[]  KbParamMax=[]  KtParamMin=[]  KtParamMax=[]  KbOutMin=[]  KbOutMax=[]  KtOutMin=[]  KtOutMax=[]  IntegratorOutMin=[]  IntegratorOutMax=[]  FilterOutMin=[]  FilterOutMax=[]  SumI1OutMin=[]  SumI1OutMax=[]  SumI2OutMin=[]  SumI2OutMax=[]  SumI3OutMin=[]  SumI3OutMax=[]  SumI4OutMin=[]  SumI4OutMax=[]  SumDOutMin=[]  SumDOutMax=[]  DifferentiatorOutMin=[]  DifferentiatorOutMax=[]  FilterDiffOutCoefMin=[]  FilterDiffOutCoefMax=[]  ReciprocalOutMin=[]  ReciprocalOutMax=[]  SumDenOutMin=[]  SumDenOutMax=[]  SumNumOutMin=[]  SumNumOutMax=[]  DivideOutMin=[]  DivideOutMax=[]  UdiffTsProdOutMin=[]  UdiffTsProdOutMax=[]  NTsProdOutMin=[]  NTsProdOutMax=[]  UintegralTsProdOutMin=[]  UintegralTsProdOutMax=[]  UngainTsProdOutMin=[]  UngainTsProdOutMax=[]  IntegratorContinuousStateAttributes=''  IntegratorStateMustResolveToSignalObject=off  IntegratorRTWStateStorageClass=Auto  FilterContinuousStateAttributes=''  FilterStateMustResolveToSignalObject=off  FilterRTWStateStorageClass=Auto  ParallelPVariant=InternalParameters  IdealPVariant=Disabled  IVariant=InternalParameters  DVariant=InternalParameters  IntegratorVariant=Continuous  SatVariant=Disabled  AWVariant=Passthrough  PCopyVariant=Disabled  TRVariant=Disabled  FdbkBlocksVariant=Forward  IdealPFdbkVariant=Disabled  SatFdbkVariant=Disabled  DerivativeFilterVariant=ContFilter  NVariant=InternalParameters  NCopyVariant=Disabled  FilterICVariant=InternalICsFilter  IntegratorICVariant=InternalICs  ExternalResetVariant=Disabled  TRSumVariant=Passthrough  SumFdbkVariant=Disabled  SumVariant=Sum_PID  TsampFilterVariant=InternalTs  TsampNgainVariant=Passthrough  TsampIntegralVariant=Passthrough  ExternalSaturationOutDataTypeStr=Inherit: Same as second input
  integrador : StateSpace  A=0  D=0  InitialCondition=InitialCondition
  motor : Subsystem
  T_m(s) : Outport
  wires:
  motor/2(omega_m(s)) -> integrador/1  "omega_m"
  Sum/1 -> controlador/1
  controlador/1 -> motor/1(Va(s))  "Va_PWM"
  theta_ref/1 -> Sum/1
  motor/1(T_m(s)) -> T_m(s)/1
  theta_m/1 -> Sum/2

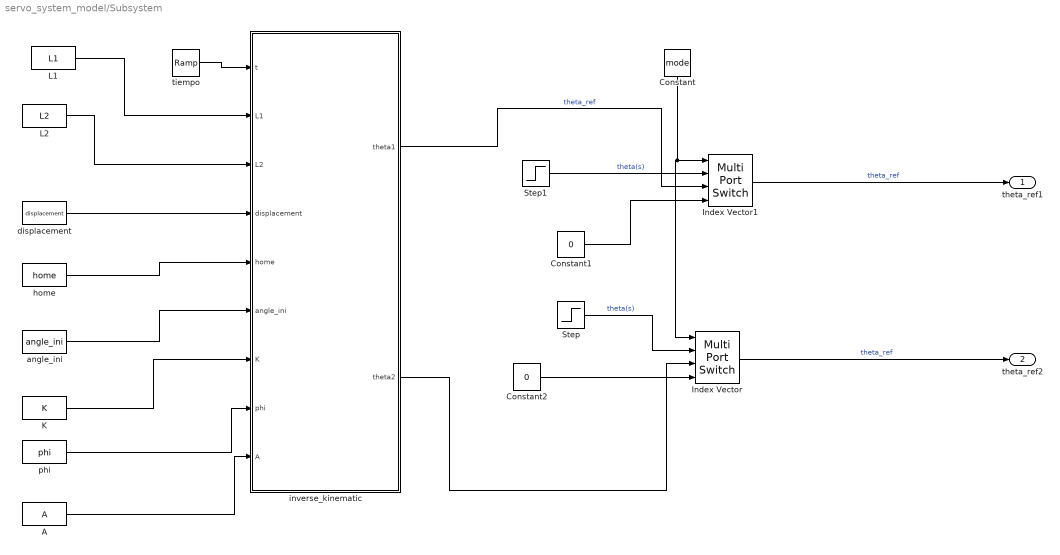
== system servo_system_model/Subsystem ==
  A : Constant  Value=A
  Constant : Constant  Value=mode
  Constant1 : Constant  Value=0
  Constant2 : Constant  Value=0
  Index Vector : MultiPortSwitch
  Index Vector1 : MultiPortSwitch
  K : Constant  Value=K
  L1 : Constant  Value=L1
  L2 : Constant  Value=L2
  Step : Step  Time=0  After=-pi/4  SampleTime=0
  Step1 : Step  Time=0  After=pi/4  SampleTime=0
  angle_ini : Constant  Value=angle_ini
  displacement : Constant  Value=displacement
  home : Constant  Value=home
  inverse_kinematic : MATLAB Function  TreatAsAtomicUnit=on
  phi : Constant  Value=phi
  tiempo : simulink/Sources/Ramp  slope=1  start=0  InitialOutput=0
  theta_ref1 : Outport
  theta_ref2 : Outport  Port=2
  wires:
  tiempo/1 -> inverse_kinematic/1(t)
  inverse_kinematic/2(theta2) -> Index Vector/3
  Constant/1 -> Index Vector/1, Index Vector1/1
  Index Vector/1 -> theta_ref2/1  "theta_ref"
  inverse_kinematic/1(theta1) -> Index Vector1/3  "theta_ref"
  Constant2/1 -> Index Vector/4
  Step/1 -> Index Vector/2  "theta(s)"
  Index Vector1/1 -> theta_ref1/1  "theta_ref"
  Constant1/1 -> Index Vector1/4
  Step1/1 -> Index Vector1/2  "theta(s)"
  angle_ini/1 -> inverse_kinematic/6(angle_ini)
  K/1 -> inverse_kinematic/7(K)
  phi/1 -> inverse_kinematic/8(phi)
  A/1 -> inverse_kinematic/9(A)
  L1/1 -> inverse_kinematic/2(L1)
  L2/1 -> inverse_kinematic/3(L2)
  displacement/1 -> inverse_kinematic/4(displacement)
  home/1 -> inverse_kinematic/5(home)

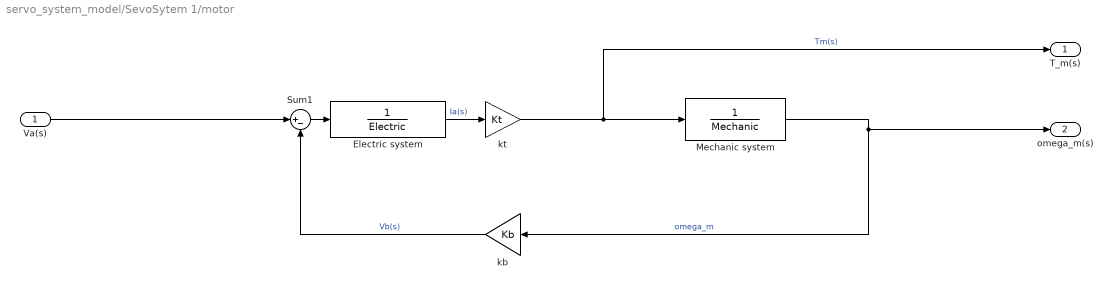
== system servo_system_model/SevoSytem 1/motor ==
  Va(s) : Inport
  Electric system : TransferFcn  Numerator=1  Denominator=Electric
  Mechanic system : TransferFcn  Numerator=1  Denominator=Mechanic
  Sum1 : Sum  Inputs=|+-
  kb : Gain  Gain=Kb
  kt : Gain  Gain=Kt
  T_m(s) : Outport
  omega_m(s) : Outport  Port=2
  wires:
  Sum1/1 -> Electric system/1
  kt/1 -> Mechanic system/1, T_m(s)/1  "Tm(s)"
  Electric system/1 -> kt/1  "Ia(s)"
  Mechanic system/1 -> omega_m(s)/1, kb/1  "omega_m"
  kb/1 -> Sum1/2  "Vb(s)"
  Va(s)/1 -> Sum1/1

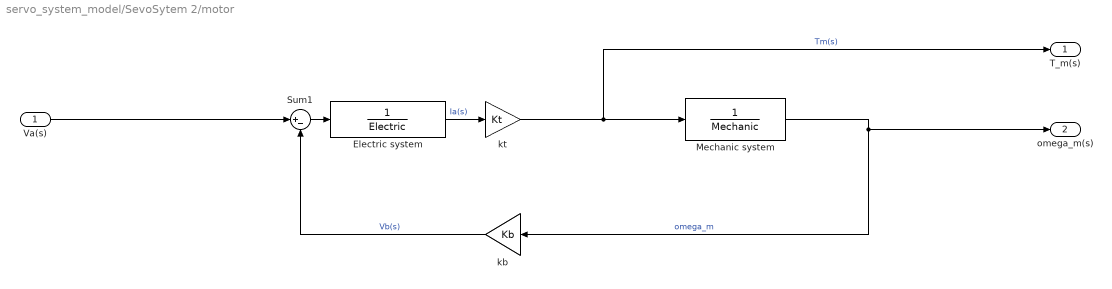
== system servo_system_model/SevoSytem 2/motor ==
  Va(s) : Inport
  Electric system : TransferFcn  Numerator=1  Denominator=Electric
  Mechanic system : TransferFcn  Numerator=1  Denominator=Mechanic
  Sum1 : Sum  Inputs=|+-
  kb : Gain  Gain=Kb
  kt : Gain  Gain=Kt
  T_m(s) : Outport
  omega_m(s) : Outport  Port=2
  wires:
  Sum1/1 -> Electric system/1
  kt/1 -> Mechanic system/1, T_m(s)/1  "Tm(s)"
  Electric system/1 -> kt/1  "Ia(s)"
  Mechanic system/1 -> omega_m(s)/1, kb/1  "omega_m"
  kb/1 -> Sum1/2  "Vb(s)"
  Va(s)/1 -> Sum1/1

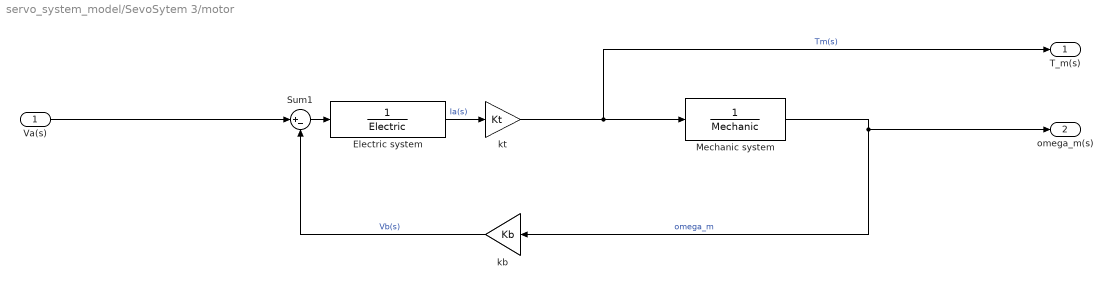
== system servo_system_model/SevoSytem 3/motor ==
  Va(s) : Inport
  Electric system : TransferFcn  Numerator=1  Denominator=Electric
  Mechanic system : TransferFcn  Numerator=1  Denominator=Mechanic
  Sum1 : Sum  Inputs=|+-
  kb : Gain  Gain=Kb
  kt : Gain  Gain=Kt
  T_m(s) : Outport
  omega_m(s) : Outport  Port=2
  wires:
  Sum1/1 -> Electric system/1
  kt/1 -> Mechanic system/1, T_m(s)/1  "Tm(s)"
  Electric system/1 -> kt/1  "Ia(s)"
  Mechanic system/1 -> omega_m(s)/1, kb/1  "omega_m"
  kb/1 -> Sum1/2  "Vb(s)"
  Va(s)/1 -> Sum1/1

== matlab function servo_system_model/Torque_g ==
  data: theta1 input; Tg1 output; Tg2 output; theta2 input
function [Tg1,Tg2]=Torque_g(theta1, theta2) 

% Distancia [cm]
L1=22;    L2=20;

% masa [kg]
m1=0.455*L1/100;   % masa barra 1
m2=0.455*L2/100;   % masa barra 2
mM1=0.2;           % masa motor 1
mM2=0.4;           % masa motor 2
mL=0.02;           % masa carga


P1=L1*R(theta1)*[1;0];
P21=L2*R(theta2+theta1)*[1;0];
P2=P21+P1;

% centro de masa 2
c2= (m2*P21/2+mL*P21)./(m2+mL);                      
% centro de masa 1
c1= (m2*(P21/2+P1) + mL*(P2+P1)+ mM2*P1 + m1*P1/2)./(m1+m2+mL+mM2);   

Tg=-9.81*[(m1+m2+mL+mM2)*c1(1);(m2+mL)*c2(1)]*10^-2;   % Torque gravitacional

Tg1=Tg(1);

Tg2=Tg(2);

  function rot=R(theta_m)
    rot=[cos(theta_m),-sin(theta_m);sin(theta_m),cos(theta_m)];
  end

end

== matlab function servo_system_model/Subsystem/inverse_kinematic ==
  data: t input; L1 input; L2 input; displacement input; home input; theta1 output; theta2 output; angle_ini input; K input; phi input; A input
function [theta1,theta2]=inverse_kinematic(t,L1,L2, displacement,home,angle_ini,K,phi,A) 

% Distancia [cm]
desp_x=displacement(1);
desp_y=displacement(2);

x_home=home(1); 
y_home=home(2);

% Parametros de trayectoria trevol estilizado
T=20;

angle=2*pi*t/T-3*pi/4;

r_base=8.5;       % radio base [cm]
K=1.1;            % factor de escala entre 1 y 1.2
phi=-3*pi/4;       % desface
A=0.4;            % factor de estilizado entre 0 y 1  
r_max=K*r_base*(1+A);

r=K*r_base*(1-A*cos(4*angle-phi));


% Desplazamiento de trayectoria
[x,y]=pol2cart(angle,r);  

x=x+desp_x;
y=y+desp_y;


[angle,r]=cart2pol(x,y);
L=sqrt(x.^2+y.^2);

% perfil de movimiento
theta=[angle-acos((L.^2+L1^2-L2^2)./(2*L*L1));
             acos((L.^2-L1^2-L2^2)/(2*L1*L2))];
theta1=theta(1);
theta2=theta(2);

end
